simulink model "single_phase_mathematical"  (R2018a)
settings: Solver=FixedStepDiscrete  StartTime=0.0  StopTime=stopTime  FixedStep=sampleTime  RelTol=1e-3
InitFcn:
  | stopTime=0.08;
  | fsw=150e3;
  | fsample=fsw*1000
  | sampleTime=1/fsample;
  | fr=fsw;
  | ffund=50;
  | m_resonant=0;
  | m_fund=0.6;
  | Lp=82e-6;
  | Ls=66e-6;
  | M=17e-6;
  | Cp=1/(4*pi*pi*Lp*fr*fr);
  | Cs=1/(4*pi*pi*Ls*fr*fr);
  | RL=40;
values from neighbouring files (symbols this model uses):
  f_fund = 50    [analytical.m]    (also in analytical2.m)
undefined symbols (not defined in the file or in its folder): Lload1, Rload1
libraries: powerlib x18, dspstat3 x1, simulink x1, powerlib_meascontrol x1
settings Model: Creator=enes_  LastModifiedBy=enes_

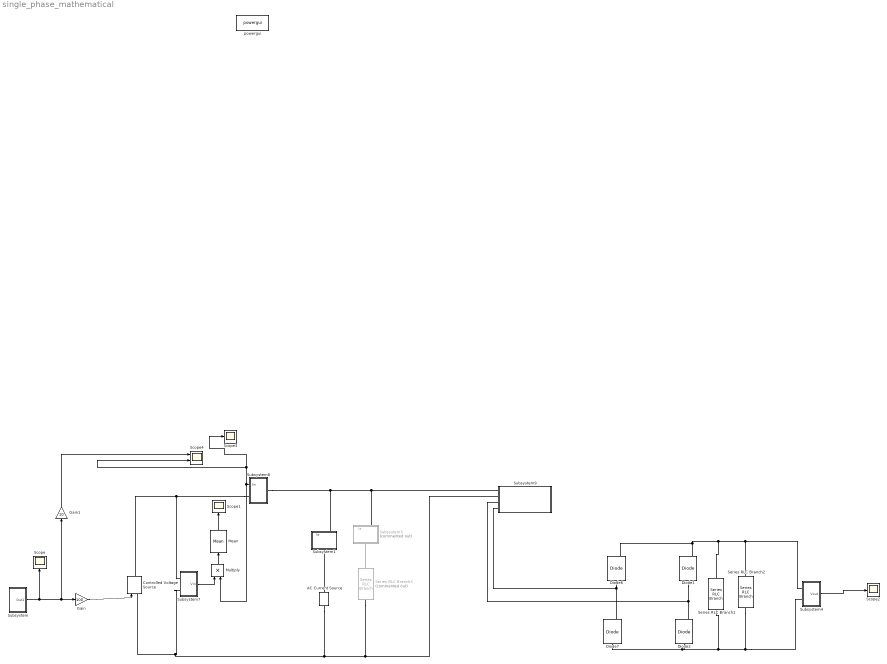
== system single_phase_mathematical ==
  AC Current Source : powerlib/Electrical Sources/AC Current Source  Amplitude=5  Phase=pi/6  Frequency=f_fund  SampleTime=0  Measurements=None
      settings: SourceProductName=Simscape Power Systems  SourceProductBaseCode=PS
  Controlled Voltage Source : powerlib/Electrical Sources/Controlled Voltage Source  Initialize=on  Source_Type=AC  Amplitude=0  Phase=0  Frequency=0  Measurements=None
  Diode{1..2,6..7} (4 alike) : powerlib/Power Electronics/Diode  Ron=0.001  Lon=0  Vf=0.8  IC=0  UseSnubber=0  Rs=500  Cs=250e-9  Measurements=on
  Gain : Gain  Gain=100
  Gain1 : Gain  Gain=10
  Mean : dspstat3/Mean  run=on  InputProcessing=Columns as channels (frame based)  reset_popup=None  directionMode=Each column  dimension=1  roiEnable=off  roiType=Rectangles  roiPortion=Entire ROI  roiOutput=Individual statistics for each ROI  roiFlag=off  roundingMode=Floor  overflowMode=off  outputDataTypeStr=Inherit: Same as accumulator  outputMin=[]  outputMax=[]  outputLastDataTypeStr=Inherit: Same as accumulator
  Multiply : Product
  Scope{,1..3} (4 alike) : Scope
  Scope4 : Scope  NumInputPorts=2
  Series RLC Branch1 : powerlib/Elements/Series RLC Branch  LConnTagsString=__new0  RConnTagsString=__new0  BranchType=C  Resistance=100e-6  Inductance=Lload1  SetiL0=off  InitialCurrent=0  Capacitance=100e-6  Setx0=off  InitialVoltage=0  Measurements=None
  Series RLC Branch2 : powerlib/Elements/Series RLC Branch  LConnTagsString=__new0  RConnTagsString=__new0  BranchType=R  Resistance=RL  Inductance=Lload1  SetiL0=off  InitialCurrent=0  Capacitance=1e-6  Setx0=off  InitialVoltage=0  Measurements=None
  Series RLC Branch3 : powerlib/Elements/Series RLC Branch  Commented=on  LConnTagsString=__new0  RConnTagsString=__new0  BranchType=RL  Resistance=10  Inductance=1e-3  SetiL0=off  InitialCurrent=0  Capacitance=1e-6  Setx0=off  InitialVoltage=0  Measurements=None
  Subsystem : Subsystem
  Subsystem1 : Subsystem
  Subsystem3 : Subsystem  Commented=on
  Subsystem4 : Subsystem
  Subsystem7 : Subsystem
  Subsystem8 : Subsystem
  Subsystem9 : Subsystem
  powergui : powerlib/powergui  Priority=1  SimulationMode=Discrete  SampleTime=sampleTime  frequency=60  Iterations=50  frequencyindice=0  Pbase=100e6  ErrMax=1e-4  UnitsV=kV  UnitsW=MW  buscounter=0  FunctionMessages=off  echomessages=off  EnableUseOfTLC=off  CurrentSourceSwitches=off  DisableSnubberDevices=off  DisableRonSwitches=off  DisableVfSwitches=off  DisplayEquations=off  SolverType=Tustin/Backward Euler (TBE)  Interpol=off  ExternalGateDelay=off  methode=off  Ts=100  x0status=blocks  SPID=on  SwTol=0  HookPort=off  RestoreLinks=warning  ResistiveCurrentMeasurement=off  Frange=[0:2:500]  Ylog=off  Xlog=on  ShowGrid=off  save=off  variable=ZData  structure=0  ZoomFFT=off  StartTime=0.0  cycles=1  DisplayStyle=1  fundamental=60  FreqAxis=off  MaxFrequency=1000  frequencyindicesteady=1  RmsSteady=1  display=off
  wires:
  Subsystem/1(Out1) -> Gain1/1, Gain/1, Scope/1
  Mean/1 -> Scope1/1
  Multiply/1 -> Mean/1
  Subsystem7/1(Vin) -> Multiply/1
  Gain/1 -> Controlled Voltage Source/1
  Subsystem4/1(Vout) -> Scope2/1
  Subsystem8/1(Iin) -> Multiply/2, Scope4/2, Scope3/1
  Gain1/1 -> Scope4/1
  connections:
  Subsystem7/LConn2 -- AC Current Source/RConn1 -- Subsystem9/LConn2 -- Series RLC Branch3/RConn1 -- Controlled Voltage Source/LConn1
  Subsystem8/RConn1 -- Controlled Voltage Source/RConn1 -- Subsystem7/LConn1
  Subsystem8/LConn1 -- Subsystem1/RConn1 -- Subsystem9/LConn1 -- Subsystem3/RConn1
  Series RLC Branch3/LConn1 -- Subsystem3/LConn1
  Diode6/LConn1 -- Subsystem9/LConn4 -- Diode7/RConn1
  Diode1/LConn1 -- Subsystem9/LConn3 -- Diode2/RConn1
  Diode7/LConn1 -- Series RLC Branch1/RConn1 -- Subsystem4/LConn2 -- Series RLC Branch2/RConn1 -- Diode2/LConn1
  Series RLC Branch2/LConn1 -- Subsystem4/LConn1 -- Series RLC Branch1/LConn1 -- Diode6/RConn1 -- Diode1/RConn1
  AC Current Source/LConn1 -- Subsystem1/LConn1

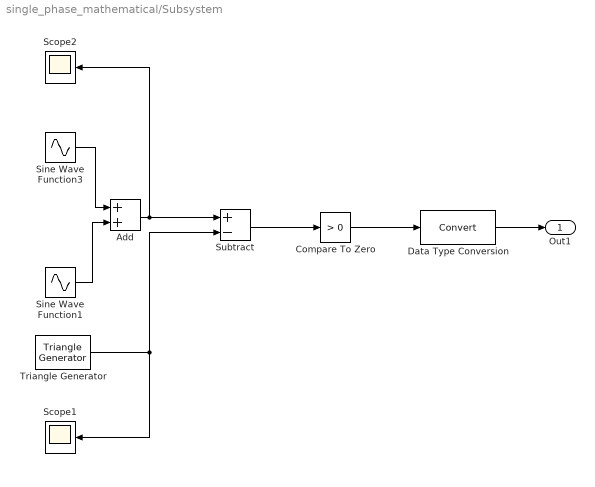
== system single_phase_mathematical/Subsystem ==
  Add : Sum
  Compare To Zero : simulink/Logic and Bit Operations/Compare To Zero  relop=>  OutDataTypeStr=boolean
  Data Type Conversion : DataTypeConversion
  Scope1 : Scope
  Scope2 : Scope
  Sine Wave Function1 : Sin  Amplitude=m_fund  Frequency=ffund*2*pi  SampleTime=0
  Sine Wave Function3 : Sin  Amplitude=m_resonant  Frequency=fr*2*pi  SampleTime=0
  Subtract : Sum  Inputs=+-
  Triangle Generator : powerlib_meascontrol/Pulse & Signal Generators/Triangle Generator  Freq=fsw  Phase=0  Ts=0
  Out1 : Outport
  wires:
  Subtract/1 -> Compare To Zero/1
  Triangle Generator/1 -> Subtract/2, Scope1/1
  Add/1 -> Subtract/1, Scope2/1
  Sine Wave Function3/1 -> Add/1
  Data Type Conversion/1 -> Out1/1
  Sine Wave Function1/1 -> Add/2
  Compare To Zero/1 -> Data Type Conversion/1

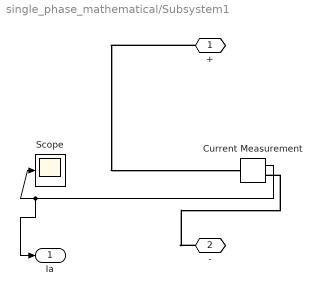
== system single_phase_mathematical/Subsystem1 ==
  Current Measurement : powerlib/Measurements/Current Measurement  PhasorSimulation=off  OutputType=Complex  PSBequivalent=0
  Scope : Scope
  + : PMIOPort  Side=Right
  - : PMIOPort  Port=2  Side=Left
  Ia : Outport
  wires:
  Current Measurement/1 -> Ia/1, Scope/1
  connections:
  +/RConn1 -- Current Measurement/LConn1
  -/RConn1 -- Current Measurement/RConn1

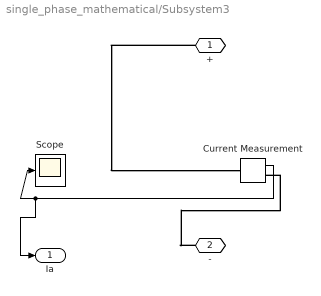
== system single_phase_mathematical/Subsystem3 ==
  Current Measurement : powerlib/Measurements/Current Measurement  PhasorSimulation=off  OutputType=Complex  PSBequivalent=0
  Scope : Scope
  + : PMIOPort  Side=Right
  - : PMIOPort  Port=2  Side=Left
  Ia : Outport
  wires:
  Current Measurement/1 -> Ia/1, Scope/1
  connections:
  +/RConn1 -- Current Measurement/LConn1
  -/RConn1 -- Current Measurement/RConn1

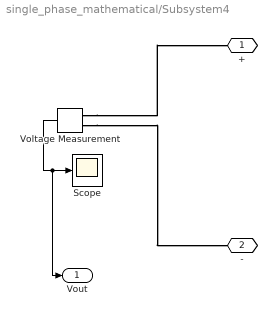
== system single_phase_mathematical/Subsystem4 ==
  Scope : Scope
  Voltage Measurement : powerlib/Measurements/Voltage Measurement  PhasorSimulation=off  OutputType=Complex  PSBequivalent=0
  + : PMIOPort  Side=Left
  - : PMIOPort  Port=2  Side=Left
  Vout : Outport
  wires:
  Voltage Measurement/1 -> Vout/1, Scope/1
  connections:
  Voltage Measurement/LConn1 -- +/RConn1
  Voltage Measurement/LConn2 -- -/RConn1

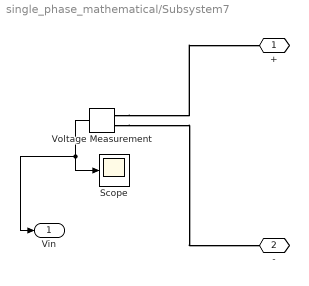
== system single_phase_mathematical/Subsystem7 ==
  Scope : Scope
  Voltage Measurement : powerlib/Measurements/Voltage Measurement  PhasorSimulation=off  OutputType=Complex  PSBequivalent=0
  + : PMIOPort  Side=Left
  - : PMIOPort  Port=2  Side=Left
  Vin : Outport
  wires:
  Voltage Measurement/1 -> Vin/1, Scope/1
  connections:
  Voltage Measurement/LConn1 -- +/RConn1
  Voltage Measurement/LConn2 -- -/RConn1

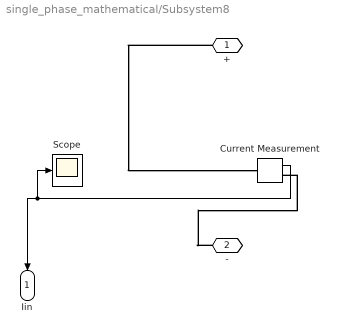
== system single_phase_mathematical/Subsystem8 ==
  Current Measurement : powerlib/Measurements/Current Measurement  PhasorSimulation=off  OutputType=Complex  PSBequivalent=0
  Scope : Scope
  + : PMIOPort  Side=Right
  - : PMIOPort  Port=2  Side=Left
  Iin : Outport
  wires:
  Current Measurement/1 -> Iin/1, Scope/1
  connections:
  +/RConn1 -- Current Measurement/LConn1
  -/RConn1 -- Current Measurement/RConn1

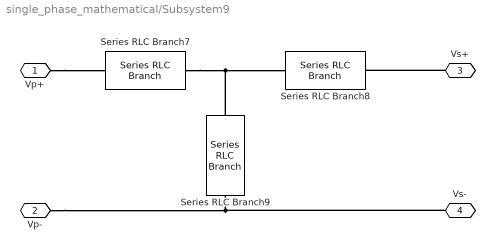
== system single_phase_mathematical/Subsystem9 ==
  Series RLC Branch7 : powerlib/Elements/Series RLC Branch  LConnTagsString=__new0  RConnTagsString=__new0  BranchType=LC  Resistance=Rload1  Inductance=Lp-M  SetiL0=off  InitialCurrent=0  Capacitance=Cp  Setx0=off  InitialVoltage=0  Measurements=None
  Series RLC Branch8 : powerlib/Elements/Series RLC Branch  LConnTagsString=__new0  RConnTagsString=__new0  BranchType=LC  Resistance=Rload1  Inductance=Ls-M  SetiL0=off  InitialCurrent=0  Capacitance=Cs  Setx0=off  InitialVoltage=0  Measurements=None
  Series RLC Branch9 : powerlib/Elements/Series RLC Branch  LConnTagsString=__new0  RConnTagsString=__new0  BranchType=L  Resistance=Rload1  Inductance=M  SetiL0=off  InitialCurrent=0  Capacitance=Cp  Setx0=off  InitialVoltage=0  Measurements=None
  Vp+ : PMIOPort  Side=Left
  Vp- : PMIOPort  Port=2  Side=Left
  Vs+ : PMIOPort  Port=3  Side=Left
  Vs- : PMIOPort  Port=4  Side=Left
  connections:
  Series RLC Branch7/LConn1 -- Series RLC Branch9/RConn1 -- Series RLC Branch8/LConn1
  Vs+/RConn1 -- Series RLC Branch8/RConn1
  Vp+/RConn1 -- Series RLC Branch7/RConn1
  Series RLC Branch9/LConn1 -- Vs-/RConn1 -- Vp-/RConn1
